simulink model "PEMFuelCellSystem_GasMixture_cEGR_RouteA_v2_v01"  (R2025b)
settings: Solver=VariableStepAuto  StartTime=0.0  StopTime=2500  RelTol=1e-3  AbsTol=1e-3
model workspace: external: MATLAB File E:\agentwork_pemfc_cEGR_0519\04_Simulink物理网络模型\01_模型\RouteA_GasMixture_Derived\PEMFuelCellSystemWithACustomLibraryParameters.m (data not in the file)
undefined symbols (not defined in the file): anode_tube_D, cathode_tube_D, cegr_valve_max_area, cegr_valve_open_min_area, comp_rpm_TLU, coolant_num_layers, coolant_num_passes, coolant_tube_D, coolant_w_channels, env_p, env_T, env_yH20, env_yO2, radiator_air_area_fins, radiator_air_area_primary, radiator_eta_fin, radiator_N_tubes, radiator_rho, radiator_t_wall, radiator_tube_H, radiator_W, routeA_air_pid_Ki, routeA_air_pid_Kp, routeA_anode_source_conditioner_nominal_flow_kg_s, routeA_cathode_source_conditioner_nominal_flow_kg_s, routeA_egr_control_Ki_area, routeA_egr_control_Kp_area, routeA_egr_target_input_mode_id, routeA_egr_valve_actuator_tau, routeA_egr_valve_area_direct, routeA_target_egr_ratio_comp_in, routeA_voltage_current_max_A, routeA_voltage_current_min_A, routeA_voltage_pi_Ki, routeA_voltage_pi_Kp, stack_area, stack_iL, stack_mea_rho, stack_num_cells, stack_num_channels, stack_t_gdl, stack_t_membrane, stack_w_channels, tank_p, tank_T, tank_yH2
libraries: FuelCell_lib x67, fl_lib x67, nesl_utility x56, slpidlib x5
(part 6 of 6)

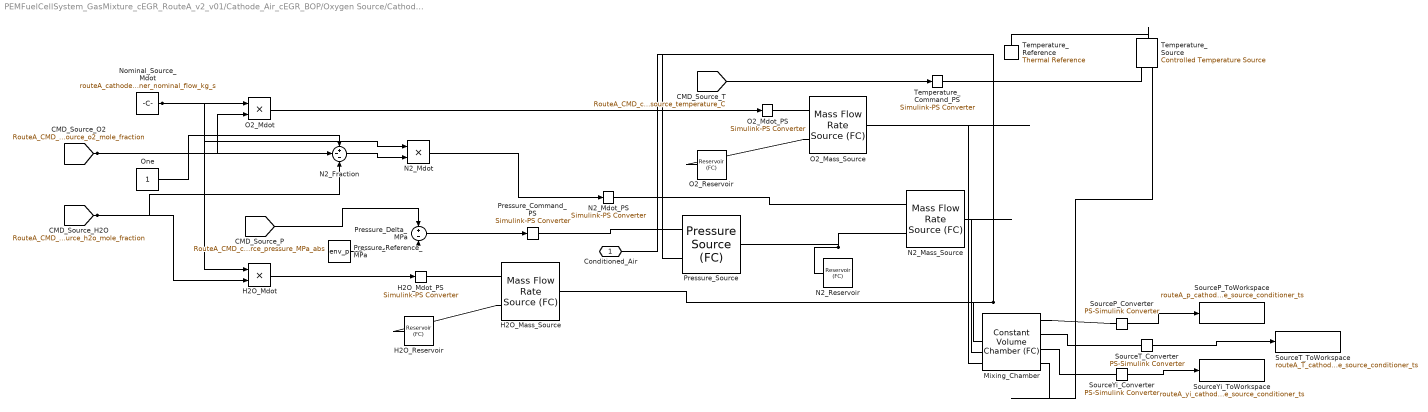
== system PEMFuelCellSystem_GasMixture_cEGR_RouteA_v2_v01/Cathode_Air_cEGR_BOP/Oxygen Source/Cathode_Source_Conditioner ==
  H2O_Mass_Source : FuelCell_lib/sources/Mass Flow Rate Source (FC)  source_type=foundation.enum.constant_controlled.controlled  flow_rate=0 kg/s  power_spec=foundation.enum.power_spec.none  area_A=0.01 m^2  area_B=0.01 m^2  mdot_A_specify=off  mdot_A_priority=None  mdot_A=0.1 kg/s  mdot_A_nominal_specify=off  mdot_A_nominal_value=1  mdot_A_nominal_unit=kg/s  mdot_B_specify=off  mdot_B_priority=None  mdot_B=0.1 kg/s  mdot_B_nominal_specify=off  mdot_B_nominal_value=1  mdot_B_nominal_unit=kg/s  phi_A_specify=off  phi_A_priority=None  phi_A=0 J/s  phi_A_nominal_specify=off  phi_A_nominal_value=1  phi_A_nominal_unit=J/s  phi_B_specify=off  phi_B_priority=None  phi_B=0 J/s  phi_B_nominal_specify=off  phi_B_nominal_value=1  phi_B_nominal_unit=J/s  mdot_A_i_specify=off  mdot_A_i_priority=None  mdot_A_i=[0; 0; 0; 0] kg/s  mdot_A_i_nominal_specify=off  mdot_A_i_nominal_value=1  mdot_A_i_nominal_unit=kg/s  mdot_B_i_specify=off  mdot_B_i_priority=None  mdot_B_i=[0; 0; 0; 0] kg/s  mdot_B_i_nominal_specify=off  mdot_B_i_nominal_value=1  mdot_B_i_nominal_unit=kg/s
      settings: InternalSimscapePortConfiguration="{\"Bottom\":[],\"Left\":[{\"id\":\"M\",\"label\":\"M\",\"type\":\"input\"},{\"id\":\"A\",\"label\":\"A\",\"type\":\"FuelCell.FuelCell\"}],\"Right\":[{\"id\":\"B\",\"label\":\"B\",\"type\":\"FuelCell.FuelCell\"}],\"Top\":[]}"
  H2O_Mdot : Product
  H2O_Mdot_PS : nesl_utility/Simulink-PS Converter  PhysicalDomain=network_engine_domain  SubClassName=ps_input  LeftPortType=input  RightPortType=output  PseudoPeriodic=off  Frequencies=[]  NoiseDistribution=none  NoiseParameters=[]  Unit=kg/s  AffineConversion=off  FilteringAndDerivatives=provide  SimscapeFilterOrder=1  InputFilterTimeConstant=0.001  UdotUserProvided=0
  H2O_Reservoir : FuelCell_lib/elements/Reservoir (FC)  constCond=true  p0=env_p * 1e6 Pa  T0=env_T + 273.15 K  comp=FuelCell.enum.Composition.Mole  y0=[0; 0; 0; 1]  x0=[0; 0; 0; 1]  area=0.01 m^2
      settings: InternalSimscapePortConfiguration="{\"Bottom\":[],\"Left\":[],\"Right\":[],\"Top\":[{\"id\":\"A\",\"label\":\"A\",\"type\":\"FuelCell.FuelCell\"}]}"
  Mixing_Chamber : FuelCell_lib/elements/Constant Volume Chamber (FC)  V0=routeA_cathode_source_conditioner_volume_L l  num_ports=foundation.enum.num_ports.three  area_A=0.01 m^2  area_B=0.01 m^2  area_C=0.01 m^2  area_D=0.01 m^2  cond_spec=FuelCell.enum.ChamberCondSpec.Enabled  tau_c=1 s  is_cond=[0; 0; 0; 1]  out_comp=FuelCell.enum.Composition.Mole  p0=env_p MPa  T0=env_T degC  comp=FuelCell.enum.Composition.Mole  y0=[1-env_yO2-env_yH20; env_yO2; 0; env_yH20]  x0=[1; 0; 0; 0]
      settings: InternalSimscapePortConfiguration="{\"Bottom\":[{\"id\":\"H\",\"label\":\"H\",\"type\":\"foundation.thermal.thermal\"}],\"Left\":[{\"id\":\"MIn\",\"label\":\"MIn\",\"type\":\"input\"},{\"id\":\"TIn\",\"label\":\"TIn\",\"type\":\"input\"}],\"Right\":[{\"id\":\"pC\",\"label\":\"p\",\"type\":\"output\"},{\"id\":\"TC\",\"label\":\"T\",\"type\":\"output\"},{\"id\":\"yC_i\",\"label\":\"y_i\",\"type\":\"output\"}],\"Top\":[{\"id\":\"A\",\"label\":\"A\",\"type\":\"FuelCell.FuelCell\"},{\"id\":\"B\",\"label\":\"B\",\"type\":\"FuelCell.FuelCell\"},{\"id\":\"C\",\"label\":\"C\",\"type\":\"FuelCell.FuelCell\"}]}"
  N2_Fraction : Sum  Inputs=+--
  N2_Mass_Source : FuelCell_lib/sources/Mass Flow Rate Source (FC)  source_type=foundation.enum.constant_controlled.controlled  flow_rate=0 kg/s  power_spec=foundation.enum.power_spec.none  area_A=0.01 m^2  area_B=0.01 m^2  mdot_A_specify=off  mdot_A_priority=None  mdot_A=0.1 kg/s  mdot_A_nominal_specify=off  mdot_A_nominal_value=1  mdot_A_nominal_unit=kg/s  mdot_B_specify=off  mdot_B_priority=None  mdot_B=0.1 kg/s  mdot_B_nominal_specify=off  mdot_B_nominal_value=1  mdot_B_nominal_unit=kg/s  phi_A_specify=off  phi_A_priority=None  phi_A=0 J/s  phi_A_nominal_specify=off  phi_A_nominal_value=1  phi_A_nominal_unit=J/s  phi_B_specify=off  phi_B_priority=None  phi_B=0 J/s  phi_B_nominal_specify=off  phi_B_nominal_value=1  phi_B_nominal_unit=J/s  mdot_A_i_specify=off  mdot_A_i_priority=None  mdot_A_i=[0; 0; 0; 0] kg/s  mdot_A_i_nominal_specify=off  mdot_A_i_nominal_value=1  mdot_A_i_nominal_unit=kg/s  mdot_B_i_specify=off  mdot_B_i_priority=None  mdot_B_i=[0; 0; 0; 0] kg/s  mdot_B_i_nominal_specify=off  mdot_B_i_nominal_value=1  mdot_B_i_nominal_unit=kg/s
      settings: InternalSimscapePortConfiguration="{\"Bottom\":[],\"Left\":[{\"id\":\"M\",\"label\":\"M\",\"type\":\"input\"},{\"id\":\"A\",\"label\":\"A\",\"type\":\"FuelCell.FuelCell\"}],\"Right\":[{\"id\":\"B\",\"label\":\"B\",\"type\":\"FuelCell.FuelCell\"}],\"Top\":[]}"
  N2_Mdot : Product
  N2_Mdot_PS : nesl_utility/Simulink-PS Converter  PhysicalDomain=network_engine_domain  SubClassName=ps_input  LeftPortType=input  RightPortType=output  PseudoPeriodic=off  Frequencies=[]  NoiseDistribution=none  NoiseParameters=[]  Unit=kg/s  AffineConversion=off  FilteringAndDerivatives=provide  SimscapeFilterOrder=1  InputFilterTimeConstant=0.001  UdotUserProvided=0
  N2_Reservoir : FuelCell_lib/elements/Reservoir (FC)  constCond=true  p0=env_p * 1e6 Pa  T0=env_T + 273.15 K  comp=FuelCell.enum.Composition.Mole  y0=[1; 0; 0; 0]  x0=[1; 0; 0; 0]  area=0.01 m^2
      settings: InternalSimscapePortConfiguration="{\"Bottom\":[],\"Left\":[],\"Right\":[],\"Top\":[{\"id\":\"A\",\"label\":\"A\",\"type\":\"FuelCell.FuelCell\"}]}"
  Nominal_Source_Mdot : Constant  Value=routeA_cathode_source_conditioner_nominal_flow_kg_s
  O2_Mass_Source : FuelCell_lib/sources/Mass Flow Rate Source (FC)  source_type=foundation.enum.constant_controlled.controlled  flow_rate=0 kg/s  power_spec=foundation.enum.power_spec.none  area_A=0.01 m^2  area_B=0.01 m^2  mdot_A_specify=off  mdot_A_priority=None  mdot_A=0.1 kg/s  mdot_A_nominal_specify=off  mdot_A_nominal_value=1  mdot_A_nominal_unit=kg/s  mdot_B_specify=off  mdot_B_priority=None  mdot_B=0.1 kg/s  mdot_B_nominal_specify=off  mdot_B_nominal_value=1  mdot_B_nominal_unit=kg/s  phi_A_specify=off  phi_A_priority=None  phi_A=0 J/s  phi_A_nominal_specify=off  phi_A_nominal_value=1  phi_A_nominal_unit=J/s  phi_B_specify=off  phi_B_priority=None  phi_B=0 J/s  phi_B_nominal_specify=off  phi_B_nominal_value=1  phi_B_nominal_unit=J/s  mdot_A_i_specify=off  mdot_A_i_priority=None  mdot_A_i=[0; 0; 0; 0] kg/s  mdot_A_i_nominal_specify=off  mdot_A_i_nominal_value=1  mdot_A_i_nominal_unit=kg/s  mdot_B_i_specify=off  mdot_B_i_priority=None  mdot_B_i=[0; 0; 0; 0] kg/s  mdot_B_i_nominal_specify=off  mdot_B_i_nominal_value=1  mdot_B_i_nominal_unit=kg/s
      settings: InternalSimscapePortConfiguration="{\"Bottom\":[],\"Left\":[{\"id\":\"M\",\"label\":\"M\",\"type\":\"input\"},{\"id\":\"A\",\"label\":\"A\",\"type\":\"FuelCell.FuelCell\"}],\"Right\":[{\"id\":\"B\",\"label\":\"B\",\"type\":\"FuelCell.FuelCell\"}],\"Top\":[]}"
  O2_Mdot : Product
  O2_Mdot_PS : nesl_utility/Simulink-PS Converter  PhysicalDomain=network_engine_domain  SubClassName=ps_input  LeftPortType=input  RightPortType=output  PseudoPeriodic=off  Frequencies=[]  NoiseDistribution=none  NoiseParameters=[]  Unit=kg/s  AffineConversion=off  FilteringAndDerivatives=provide  SimscapeFilterOrder=1  InputFilterTimeConstant=0.001  UdotUserProvided=0
  O2_Reservoir : FuelCell_lib/elements/Reservoir (FC)  constCond=true  p0=env_p * 1e6 Pa  T0=env_T + 273.15 K  comp=FuelCell.enum.Composition.Mole  y0=[0; 1; 0; 0]  x0=[0; 1; 0; 0]  area=0.01 m^2
      settings: InternalSimscapePortConfiguration="{\"Bottom\":[],\"Left\":[],\"Right\":[],\"Top\":[{\"id\":\"A\",\"label\":\"A\",\"type\":\"FuelCell.FuelCell\"}]}"
  One : Constant
  Pressure_Command_PS : nesl_utility/Simulink-PS Converter  PhysicalDomain=network_engine_domain  SubClassName=ps_input  LeftPortType=input  RightPortType=output  PseudoPeriodic=off  Frequencies=[]  NoiseDistribution=none  NoiseParameters=[]  Unit=MPa  AffineConversion=off  FilteringAndDerivatives=filter  SimscapeFilterOrder=1  InputFilterTimeConstant=0.001  UdotUserProvided=0
  Pressure_Delta_MPa : Sum  Inputs=+-
  Pressure_Reference_MPa : Constant  Value=env_p
  Pressure_Source : FuelCell_lib/sources/Pressure Source (FC)  source_type=foundation.enum.constant_controlled.controlled  pressure_differential=0 Pa  power_spec=foundation.enum.power_spec.none  area_A=0.01 m^2  area_B=0.01 m^2  mdot_A_specify=off  mdot_A_priority=None  mdot_A=0.1 kg/s  mdot_A_nominal_specify=off  mdot_A_nominal_value=1  mdot_A_nominal_unit=kg/s  mdot_B_specify=off  mdot_B_priority=None  mdot_B=0.1 kg/s  mdot_B_nominal_specify=off  mdot_B_nominal_value=1  mdot_B_nominal_unit=kg/s  phi_A_specify=off  phi_A_priority=None  phi_A=0 J/s  phi_A_nominal_specify=off  phi_A_nominal_value=1  phi_A_nominal_unit=J/s  phi_B_specify=off  phi_B_priority=None  phi_B=0 J/s  phi_B_nominal_specify=off  phi_B_nominal_value=1  phi_B_nominal_unit=J/s  mdot_A_i_specify=off  mdot_A_i_priority=None  mdot_A_i=[0; 0; 0; 0] kg/s  mdot_A_i_nominal_specify=off  mdot_A_i_nominal_value=1  mdot_A_i_nominal_unit=kg/s  mdot_B_i_specify=off  mdot_B_i_priority=None  mdot_B_i=[0; 0; 0; 0] kg/s  mdot_B_i_nominal_specify=off  mdot_B_i_nominal_value=1  mdot_B_i_nominal_unit=kg/s
      settings: InternalSimscapePortConfiguration="{\"Bottom\":[],\"Left\":[{\"id\":\"p\",\"label\":\"P\",\"type\":\"input\"},{\"id\":\"A\",\"label\":\"A\",\"type\":\"FuelCell.FuelCell\"}],\"Right\":[{\"id\":\"B\",\"label\":\"B\",\"type\":\"FuelCell.FuelCell\"}],\"Top\":[]}"
  SourceP_Converter : nesl_utility/PS-Simulink Converter  PhysicalDomain=network_engine_domain  SubClassName=ps_output  LeftPortType=input  RightPortType=output  PseudoPeriodic=off  Frequencies=[]  VectorFormat=inherit  Unit=inherit  AffineConversion=off
  SourceP_ToWorkspace : ToWorkspace  VariableName=routeA_p_cathode_source_conditioner_ts  SaveFormat=Timeseries  SampleTime=-1
  SourceT_Converter : nesl_utility/PS-Simulink Converter  PhysicalDomain=network_engine_domain  SubClassName=ps_output  LeftPortType=input  RightPortType=output  PseudoPeriodic=off  Frequencies=[]  VectorFormat=inherit  Unit=inherit  AffineConversion=off
  SourceT_ToWorkspace : ToWorkspace  VariableName=routeA_T_cathode_source_conditioner_ts  SaveFormat=Timeseries  SampleTime=-1
  SourceYi_Converter : nesl_utility/PS-Simulink Converter  PhysicalDomain=network_engine_domain  SubClassName=ps_output  LeftPortType=input  RightPortType=output  PseudoPeriodic=off  Frequencies=[]  VectorFormat=inherit  Unit=inherit  AffineConversion=off
  SourceYi_ToWorkspace : ToWorkspace  VariableName=routeA_yi_cathode_source_conditioner_ts  SaveFormat=Timeseries  SampleTime=-1
  Temperature_Command_PS : nesl_utility/Simulink-PS Converter  PhysicalDomain=network_engine_domain  SubClassName=ps_input  LeftPortType=input  RightPortType=output  PseudoPeriodic=off  Frequencies=[]  NoiseDistribution=none  NoiseParameters=[]  Unit=degC  AffineConversion=off  FilteringAndDerivatives=filter  SimscapeFilterOrder=1  InputFilterTimeConstant=0.001  UdotUserProvided=0
  Temperature_Reference : fl_lib/Thermal/Thermal Elements/Thermal Reference
  Temperature_Source : fl_lib/Thermal/Thermal Sources/Controlled Temperature Source
  Conditioned_Air : PMIOPort  Side=Right
  wires:
  SourceYi_Converter/1 -> SourceYi_ToWorkspace/1
  SourceT_Converter/1 -> SourceT_ToWorkspace/1
  Pressure_Delta_MPa/1 -> Pressure_Command_PS/1
  Pressure_Reference_MPa/1 -> Pressure_Delta_MPa/2
  [RouteA_CMD_cathode_source_pressure_MPa_abs] -> Pressure_Delta_MPa/1
  [RouteA_CMD_cathode_source_temperature_C] -> Temperature_Command_PS/1
  One/1 -> N2_Fraction/1
  [RouteA_CMD_cathode_source_o2_mole_fraction] -> O2_Mdot/2, N2_Fraction/2
  [RouteA_CMD_cathode_source_h2o_mole_fraction] -> N2_Fraction/3, H2O_Mdot/2
  Nominal_Source_Mdot/1 -> O2_Mdot/1, N2_Mdot/1, H2O_Mdot/1
  N2_Fraction/1 -> N2_Mdot/2
  N2_Mdot/1 -> N2_Mdot_PS/1
  O2_Mdot/1 -> O2_Mdot_PS/1
  H2O_Mdot/1 -> H2O_Mdot_PS/1
  SourceP_Converter/1 -> SourceP_ToWorkspace/1
  connections:
  Mixing_Chamber/RConn3 -- SourceYi_Converter/LConn1
  Mixing_Chamber/RConn2 -- SourceT_Converter/LConn1
  Pressure_Command_PS/RConn1 -- Pressure_Source/LConn1
  Mixing_Chamber/LConn3 -- H2O_Mass_Source/RConn1 -- Pressure_Source/LConn2 -- Conditioned_Air/RConn1
  Temperature_Command_PS/RConn1 -- Temperature_Source/RConn1
  Temperature_Source/RConn2 -- Mixing_Chamber/RConn4
  Temperature_Source/LConn1 -- Temperature_Reference/LConn1
  N2_Mdot_PS/RConn1 -- N2_Mass_Source/LConn1
  O2_Mdot_PS/RConn1 -- O2_Mass_Source/LConn1
  H2O_Mdot_PS/RConn1 -- H2O_Mass_Source/LConn1
  N2_Reservoir/LConn1 -- Pressure_Source/RConn1 -- N2_Mass_Source/LConn2
  O2_Reservoir/LConn1 -- O2_Mass_Source/LConn2
  H2O_Reservoir/LConn1 -- H2O_Mass_Source/LConn2
  N2_Mass_Source/RConn1 -- Mixing_Chamber/LConn4
  O2_Mass_Source/RConn1 -- Mixing_Chamber/LConn5
  Mixing_Chamber/RConn1 -- SourceP_Converter/LConn1

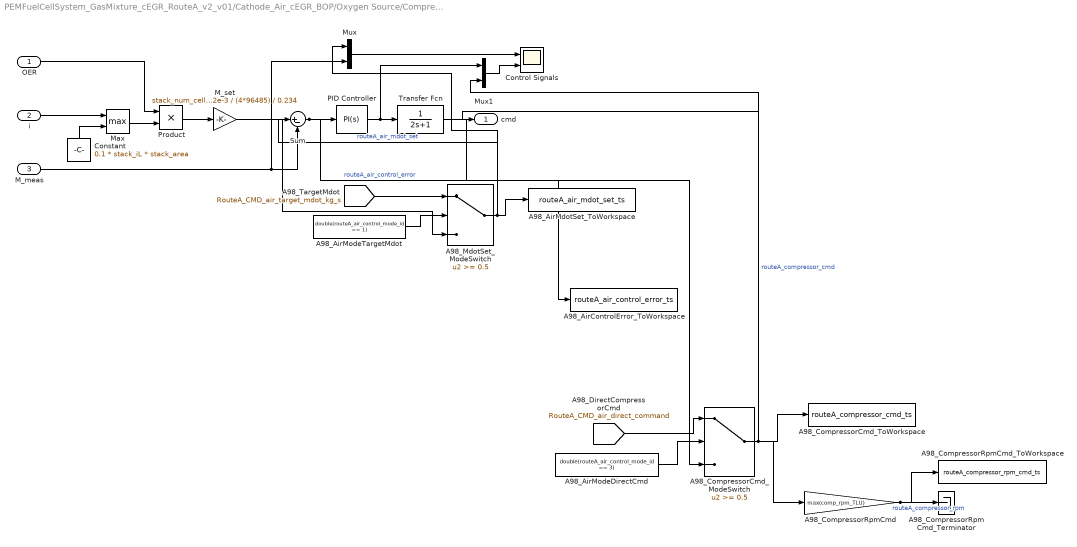
== system PEMFuelCellSystem_GasMixture_cEGR_RouteA_v2_v01/Cathode_Air_cEGR_BOP/Oxygen Source/Compressor Control ==
  OER : Inport
  i : Inport  Port=2
  M_meas : Inport  Port=3
  A98_AirControlError_ToWorkspace : ToWorkspace  VariableName=routeA_air_control_error_ts  SaveFormat=Timeseries  SampleTime=-1
  A98_AirMdotSet_ToWorkspace : ToWorkspace  VariableName=routeA_air_mdot_set_ts  SaveFormat=Timeseries  SampleTime=-1
  A98_AirModeDirectCmd : Constant  Value=double(routeA_air_control_mode_id == 3)
  A98_AirModeTargetMdot : Constant  Value=double(routeA_air_control_mode_id == 1)
  A98_CompressorCmd_ModeSwitch : Switch  Threshold=0.5  SaturateOnIntegerOverflow=off  InputSameDT=off
  A98_CompressorCmd_ToWorkspace : ToWorkspace  VariableName=routeA_compressor_cmd_ts  SaveFormat=Timeseries  SampleTime=-1
  A98_CompressorRpmCmd : Gain  Gain=max(comp_rpm_TLU)
  A98_CompressorRpmCmd_Terminator : Terminator
  A98_CompressorRpmCmd_ToWorkspace : ToWorkspace  VariableName=routeA_compressor_rpm_cmd_ts  SaveFormat=Timeseries  SampleTime=-1
  A98_MdotSet_ModeSwitch : Switch  Threshold=0.5  SaturateOnIntegerOverflow=off  InputSameDT=off
  Constant : Constant  Value=0.1 * stack_iL * stack_area
  Control Signals : Scope  NumInputPorts=2
      settings: Title=Mass Flow Rate (kg/s)  ActiveDisplayYMinimum=-0.01736  ActiveDisplayYMaximum=0.15625  DataLoggingVariableName=ScopeData2
  M_set : Gain  Gain=stack_num_cells * 32e-3 / (4*96485) / 0.234
  Max : MinMax  Function=max  Inputs=2  ZeroCross=off
  Mux : Mux  Inputs=2
  Mux1 : Mux  Inputs=2
  PID Controller : slpidlib/PID Controller  Controller=PI  Form=Ideal  TimeDomain=Continuous-time  UseExternalTs=off  SampleTime=-1  IntegratorMethod=Forward Euler  FilterMethod=Forward Euler  ControllerParametersSource=internal  P=routeA_air_pid_Kp  I=routeA_air_pid_Ki  UseKiTs=off  D=0  UseExternalDerivativeSource=off  N=100  UseFilter=on  TunerSelectOption=Transfer Function Based (PID Tuner App)  InitialConditionSource=internal  InitialConditionForIntegrator=0  InitialConditionForFilter=0  DifferentiatorICPrevScaledInput=0  ExternalReset=none  TrackingMode=off  Kt=1  LimitOutput=on  SatLimitsSource=internal  UpperSaturationLimit=1  LowerSaturationLimit=0  LinearizeAsGain=on  AntiWindupMode=back-calculation  Kb=1  LimitIntegrator=off  UpperIntegratorSaturationLimit=inf  LowerIntegratorSaturationLimit=-inf  POutMin=[]  POutMax=[]  IOutMin=[]  IOutMax=[]  DOutMin=[]  DOutMax=[]  NOutMin=[]  NOutMax=[]  SumOutMin=[]  SumOutMax=[]  SaturationOutMin=[]  SaturationOutMax=[]  PParamMin=[]  PParamMax=[]  IParamMin=[]  IParamMax=[]  DParamMin=[]  DParamMax=[]  NParamMin=[]  NParamMax=[]  KbParamMin=[]  KbParamMax=[]  KtParamMin=[]  KtParamMax=[]  KbOutMin=[]  KbOutMax=[]  KtOutMin=[]  KtOutMax=[]  IntegratorOutMin=[]  IntegratorOutMax=[]  FilterOutMin=[]  FilterOutMax=[]  SumI1OutMin=[]  SumI1OutMax=[]  SumI2OutMin=[]  SumI2OutMax=[]  SumI3OutMin=[]  SumI3OutMax=[]  SumI4OutMin=[]  SumI4OutMax=[]  SumDOutMin=[]  SumDOutMax=[]  DifferentiatorOutMin=[]  DifferentiatorOutMax=[]  FilterDiffOutCoefMin=[]  FilterDiffOutCoefMax=[]  ReciprocalOutMin=[]  ReciprocalOutMax=[]  SumDenOutMin=[]  SumDenOutMax=[]  SumNumOutMin=[]  SumNumOutMax=[]  DivideOutMin=[]  DivideOutMax=[]  UdiffTsProdOutMin=[]  UdiffTsProdOutMax=[]  NTsProdOutMin=[]  NTsProdOutMax=[]  UintegralTsProdOutMin=[]  UintegralTsProdOutMax=[]  UngainTsProdOutMin=[]  UngainTsProdOutMax=[]  ClampingZeroOutDataTypeStr=Inherit: Inherit via back propagation  ClampingZeroOutMin=[]  ClampingZeroOutMax=[]  FilterDenConstantOutDataTypeStr=Inherit: Inherit via back propagation  FilterDenConstantOutMin=[]  FilterDenConstantOutMax=[]  PCopyOutDataTypeStr=Inherit: Inherit via back propagation  PCopyOutMin=[]  PCopyOutMax=[]  NCopyOutDataTypeStr=Inherit: Inherit via back propagation  NCopyOutMin=[]  NCopyOutMax=[]  IntegratorContinuousStateAttributes=''  IntegratorStateMustResolveToSignalObject=off  IntegratorRTWStateStorageClass=Auto  FilterContinuousStateAttributes=''  FilterStateMustResolveToSignalObject=off  FilterRTWStateStorageClass=Auto  ParallelPVariant=Passthrough  IdealPVariant=InternalParameters  IVariant=InternalParameters  DVariant=Disabled  IntegratorVariant=Continuous  SatVariant=Enabled  AWVariant=BackCalculation  PCopyVariant=Disabled  TRVariant=Disabled  FdbkBlocksVariant=Forward  IdealPFdbkVariant=Disabled  SatFdbkVariant=Disabled  DerivativeFilterVariant=Disabled  NVariant=Disabled  NCopyVariant=Disabled_SignalSpec  FilterICVariant=Disabled  IntegratorICVariant=InternalICs  ExternalResetVariant=Disabled  TRSumVariant=Passthrough  SumFdbkVariant=Disabled  SumVariant=Sum_PI  TsampFilterVariant=InternalTs  TsampNgainVariant=Passthrough  TsampIntegralVariant=Disabled_SignalSpec  ExternalSaturationOutDataTypeStr=Inherit: Same as second input  DerivativeSourceVariant=Disabled  PreIntVariant=InternalPreInt
  Product : Product
  Sum : Sum  Inputs=|+-
  Transfer Fcn : TransferFcn  Denominator=[2 1]
  cmd : Outport
  wires:
  OER/1 -> Product/1
  Constant/1 -> Max/2
  i/1 -> Max/1
  Max/1 -> Product/2
  PID Controller/1 -> Mux1/1, Transfer Fcn/1
  Sum/1 -> PID Controller/1, A98_AirControlError_ToWorkspace/1  "routeA_air_control_error"
  Product/1 -> M_set/1
  M_meas/1 -> Mux/2, Sum/2
  Mux/1 -> Control Signals/1
  Mux1/1 -> Control Signals/2
  A98_AirModeTargetMdot/1 -> A98_MdotSet_ModeSwitch/2
  M_set/1 -> A98_MdotSet_ModeSwitch/3
  A98_MdotSet_ModeSwitch/1 -> Sum/1, Mux/1, A98_AirMdotSet_ToWorkspace/1  "routeA_air_mdot_set"
  A98_AirModeDirectCmd/1 -> A98_CompressorCmd_ModeSwitch/2
  Transfer Fcn/1 -> A98_CompressorCmd_ModeSwitch/3
  A98_CompressorCmd_ModeSwitch/1 -> cmd/1, Mux1/2, A98_CompressorRpmCmd/1, A98_CompressorCmd_ToWorkspace/1  "routeA_compressor_cmd"
  A98_CompressorRpmCmd/1 -> A98_CompressorRpmCmd_Terminator/1, A98_CompressorRpmCmd_ToWorkspace/1  "routeA_compressor_rpm"
  [RouteA_CMD_air_target_mdot_kg_s] -> A98_MdotSet_ModeSwitch/1
  [RouteA_CMD_air_direct_command] -> A98_CompressorCmd_ModeSwitch/1

== system PEMFuelCellSystem_GasMixture_cEGR_RouteA_v2_v01/Cathode_Air_cEGR_BOP/Oxygen Source/Compressor Map ==
  1 / 101325 : fl_lib/Physical Signals/Functions/PS Gain  gain=1 / 101325 1/Pa
  1 / 288.15 : fl_lib/Physical Signals/Functions/PS Gain  gain=1 / 288.15 1/K
  Absolute Reference (FC) : FuelCell_lib/elements/Absolute Reference (FC)
      settings: InternalSimscapePortConfiguration="{\"Bottom\":[],\"Left\":[{\"id\":\"A\",\"label\":\"\",\"type\":\"FuelCell.FuelCell\"}],\"Right\":[],\"Top\":[]}"
  Absolute Reference (FC)1 : FuelCell_lib/elements/Absolute Reference (FC)
      settings: InternalSimscapePortConfiguration="{\"Bottom\":[],\"Left\":[{\"id\":\"A\",\"label\":\"\",\"type\":\"FuelCell.FuelCell\"}],\"Right\":[],\"Top\":[]}"
  Corrected Flow Table : fl_lib/Physical Signals/Lookup Tables/PS Lookup Table (2D)  x1=comp_p_ratio_TLU Pa/Pa  x2=comp_rpm_TLU rpm  f=comp_mdot_corr_TLU kg/s  interp_method=simscape.enum.interpolation.linear  extrap_method=simscape.enum.extrapolation.nearest
  PS Divide : fl_lib/Physical Signals/Functions/PS Divide
  PS Divide1 : fl_lib/Physical Signals/Functions/PS Divide
  PS Product : fl_lib/Physical Signals/Functions/PS Product
  Pressure and Temperature Sensor (FC) : FuelCell_lib/sensors/Pressure and Temperature Sensor (FC)
      settings: InternalSimscapePortConfiguration="{\"Bottom\":[],\"Left\":[{\"id\":\"A\",\"label\":\"A\",\"type\":\"FuelCell.FuelCell\"}],\"Right\":[{\"id\":\"P\",\"label\":\"P\",\"type\":\"output\"},{\"id\":\"T\",\"label\":\"T\",\"type\":\"output\"},{\"id\":\"B\",\"label\":\"B\",\"type\":\"FuelCell.FuelCell\"}],\"Top\":[]}"
  Pressure and Temperature Sensor (FC)1 : FuelCell_lib/sensors/Pressure and Temperature Sensor (FC)
      settings: InternalSimscapePortConfiguration="{\"Bottom\":[],\"Left\":[{\"id\":\"A\",\"label\":\"A\",\"type\":\"FuelCell.FuelCell\"}],\"Right\":[{\"id\":\"P\",\"label\":\"P\",\"type\":\"output\"},{\"id\":\"T\",\"label\":\"T\",\"type\":\"output\"},{\"id\":\"B\",\"label\":\"B\",\"type\":\"FuelCell.FuelCell\"}],\"Top\":[]}"
  TDenGuardBias : fl_lib/Physical Signals/Functions/PS Bias  bias=cegr_comp_map_t_denom_epsilon
      settings: InternalSimscapePortConfiguration="{\"Bottom\":[],\"Left\":[{\"id\":\"I\",\"label\":\"\",\"type\":\"input\"}],\"Right\":[{\"id\":\"O\",\"label\":\"\",\"type\":\"output\"}],\"Top\":[]}"
  sqrt : fl_lib/Physical Signals/Functions/PS Math Function  fcn_choice=foundation.enum.math_function.sqrt  v=1
  mdot : PMIOPort  Side=Left
  in : PMIOPort  Port=2  Side=Right
  rpm : PMIOPort  Port=3  Side=Right
  out : PMIOPort  Port=4  Side=Right
  connections:
  1 / 101325/LConn1 -- Pressure and Temperature Sensor (FC)/RConn1 -- PS Divide/LConn2
  rpm/RConn1 -- Corrected Flow Table/LConn2
  PS Divide/RConn1 -- Corrected Flow Table/LConn1
  1 / 288.15/LConn1 -- Pressure and Temperature Sensor (FC)/RConn2
  PS Product/LConn1 -- 1 / 101325/RConn1
  PS Product/LConn2 -- Corrected Flow Table/RConn1
  PS Divide1/LConn1 -- PS Product/RConn1
  1 / 288.15/RConn1 -- sqrt/LConn1
  mdot/RConn1 -- PS Divide1/RConn1
  Pressure and Temperature Sensor (FC)1/RConn1 -- PS Divide/LConn1
  Absolute Reference (FC)/LConn1 -- Pressure and Temperature Sensor (FC)/RConn3
  Pressure and Temperature Sensor (FC)/LConn1 -- in/RConn1
  Absolute Reference (FC)1/LConn1 -- Pressure and Temperature Sensor (FC)1/RConn3
  Pressure and Temperature Sensor (FC)1/LConn1 -- out/RConn1
  sqrt/RConn1 -- TDenGuardBias/LConn1
  TDenGuardBias/RConn1 -- PS Divide1/LConn2

== system PEMFuelCellSystem_GasMixture_cEGR_RouteA_v2_v01/Cathode_Exhaust_Backpressure_Water/Cathode Exhaust/Pressure Relief Valve ==
  Absolute Reference (FC) : FuelCell_lib/elements/Absolute Reference (FC)
      settings: InternalSimscapePortConfiguration="{\"Bottom\":[],\"Left\":[{\"id\":\"A\",\"label\":\"\",\"type\":\"FuelCell.FuelCell\"}],\"Right\":[],\"Top\":[]}"
  PS Add : fl_lib/Physical Signals/Functions/PS Add
  PS Constant : fl_lib/Physical Signals/Sources/PS Constant  constant=r_min^2
  PS Gain : fl_lib/Physical Signals/Functions/PS Gain  gain=(r_max^2 - r_min^2)/p_range 1/MPa
  PS Gain1 : fl_lib/Physical Signals/Functions/PS Gain  gain=pi*D^2/4 m^2
  PS Subtract : fl_lib/Physical Signals/Functions/PS Subtract
  Pressure and Temperature Sensor (FC) : FuelCell_lib/sensors/Pressure and Temperature Sensor (FC)
      settings: InternalSimscapePortConfiguration="{\"Bottom\":[],\"Left\":[{\"id\":\"A\",\"label\":\"A\",\"type\":\"FuelCell.FuelCell\"}],\"Right\":[{\"id\":\"P\",\"label\":\"P\",\"type\":\"output\"},{\"id\":\"T\",\"label\":\"T\",\"type\":\"output\"},{\"id\":\"B\",\"label\":\"B\",\"type\":\"FuelCell.FuelCell\"}],\"Top\":[]}"
  Valve : FuelCell_lib/elements/Local Restriction (FC)  const_area=false  restriction_area=0.001 m^2  min_area=pi*(r_min*D)^2/4 m^2  max_area=pi*(r_max*D)^2/4 m^2  area=pi*D^2/4 m^2  Cd=0.64  B_lam=0.999
      settings: InternalSimscapePortConfiguration="{\"Bottom\":[],\"Left\":[{\"id\":\"AR\",\"label\":\"AR\",\"type\":\"input\"},{\"id\":\"A\",\"label\":\"A\",\"type\":\"FuelCell.FuelCell\"}],\"Right\":[{\"id\":\"B\",\"label\":\"B\",\"type\":\"FuelCell.FuelCell\"}],\"Top\":[]}"
  A : PMIOPort  Side=Left
  B : PMIOPort  Port=2  Side=Right
  p_set : PMIOPort  Port=3  Side=Left
  connections:
  PS Add/RConn1 -- PS Gain1/LConn1
  PS Gain/LConn1 -- PS Subtract/RConn1
  PS Gain1/RConn1 -- Valve/LConn1
  Valve/RConn1 -- B/RConn1
  A/RConn1 -- Pressure and Temperature Sensor (FC)/LConn1 -- Valve/LConn2
  PS Gain/RConn1 -- PS Add/LConn1
  PS Add/LConn2 -- PS Constant/RConn1
  p_set/RConn1 -- PS Subtract/LConn2
  Pressure and Temperature Sensor (FC)/RConn1 -- PS Subtract/LConn1
  Absolute Reference (FC)/LConn1 -- Pressure and Temperature Sensor (FC)/RConn3

== system PEMFuelCellSystem_GasMixture_cEGR_RouteA_v2_v01/System_Control_Observability/Electrical Load/Inputs ==
  Current Demand : Subsystem  VariantControl=Current
      settings: PortSchema="{\"entries\":[{\"content\":{\"sides\":[{\"content\":{\"connectorIds\":[\"LConn1\"]},\"type\":\"ConnectorPlacement.EquallySpacedRectSide\",\"uuid\":\"316ab41f-9548-4c29-941b-82cd3006a9cc\"},{\"content\":{\"connectorIds\":[],\"side\":\"RIGHT\"},\"type\":\"ConnectorPlacement.EquallySpacedRectSide\",\"uuid\":\"21ddf6a1-5f8a-47a4-ab15-3c27c3a556ce\"},{\"content\":{\"connectorIds\":[\"LConn2\"],\"side\":\"TOP\"},\"type\":\"ConnectorPlacement.EquallySpacedRectSide\",\"uuid\":\"59191a52-f145-4ac2-9cf2-0e0b54b3d2a8\"}]},\"type\":\"ConnectorPlacement.EquallySpacedConnector\",\"uuid\":\"e8f988fd-b412-4b1a-aaea-374cf82170cc\"}],\"packageUris\":[\"http://schema.mathworks.com/mf0/Connector/R2020b\"],\"version\":\"1.0\"}"
      mask Display:
      | plot(0, 0)
      | plot(100, 100)
      | 
      | plot([20 50 50 80], [20 20 80 80])
  Power Demand : Subsystem  VariantControl=Power
      settings: PortSchema="{\"entries\":[{\"content\":{\"sides\":[{\"content\":{\"connectorIds\":[\"LConn1\"]},\"type\":\"ConnectorPlacement.EquallySpacedRectSide\",\"uuid\":\"316ab41f-9548-4c29-941b-82cd3006a9cc\"},{\"content\":{\"connectorIds\":[],\"side\":\"RIGHT\"},\"type\":\"ConnectorPlacement.EquallySpacedRectSide\",\"uuid\":\"21ddf6a1-5f8a-47a4-ab15-3c27c3a556ce\"},{\"content\":{\"connectorIds\":[\"LConn2\"],\"side\":\"TOP\"},\"type\":\"ConnectorPlacement.EquallySpacedRectSide\",\"uuid\":\"59191a52-f145-4ac2-9cf2-0e0b54b3d2a8\"}]},\"type\":\"ConnectorPlacement.EquallySpacedConnector\",\"uuid\":\"e8f988fd-b412-4b1a-aaea-374cf82170cc\"}],\"packageUris\":[\"http://schema.mathworks.com/mf0/Connector/R2020b\"],\"version\":\"1.0\"}"
      mask Display:
      | plot(0, 0)
      | plot(100, 100)
      | 
      | mws = get_param(bdroot, 'ModelWorkspace');
      | x = getVariable(mws, 'drive_cycle_time');
      | y = getVariable(mws, 'drive_cycle_power');
      | 
      | plot(x/max(x)*80 + 10, y/max(y)*60 + 30)
  Voltage Demand : Subsystem  VariantControl=Voltage
  i : PMIOPort  Side=Left
  v : PMIOPort  Port=2  Side=Left

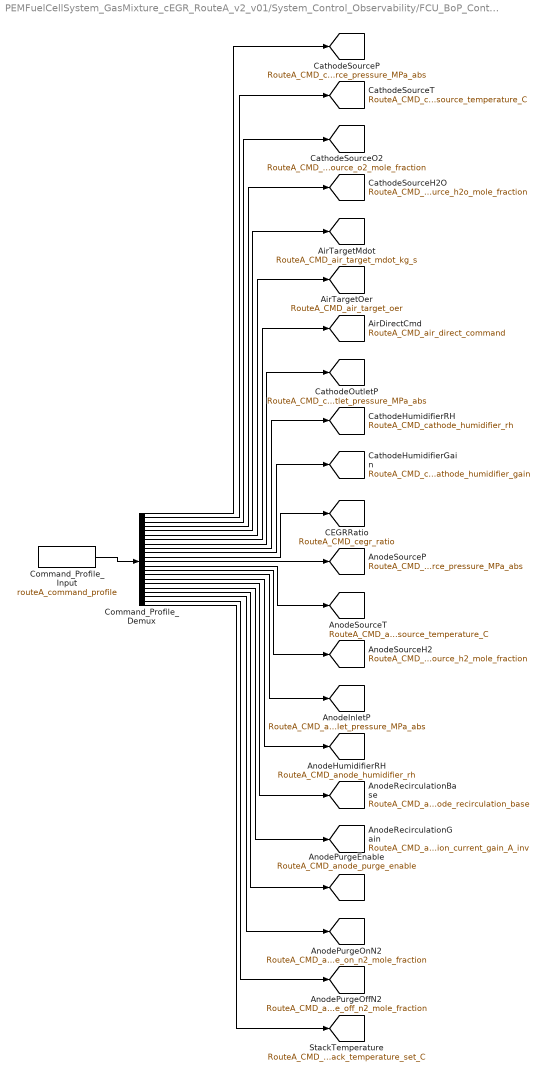
== system PEMFuelCellSystem_GasMixture_cEGR_RouteA_v2_v01/System_Control_Observability/FCU_BoP_Control/RouteA_Command_Profile ==
  Command_Profile_Demux : Demux  Outputs=22
  Command_Profile_Input : FromWorkspace  VariableName=routeA_command_profile  OutputAfterFinalValue=Holding final value
  tag scope: RouteA_CMD_air_direct_command=global, RouteA_CMD_air_target_mdot_kg_s=global, RouteA_CMD_air_target_oer=global, RouteA_CMD_anode_humidifier_rh=global, RouteA_CMD_anode_inlet_pressure_MPa_abs=global, RouteA_CMD_anode_purge_enable=global, RouteA_CMD_anode_purge_off_n2_mole_fraction=global, RouteA_CMD_anode_purge_on_n2_mole_fraction=global, RouteA_CMD_anode_recirculation_base=global, RouteA_CMD_anode_recirculation_current_gain_A_inv=global, RouteA_CMD_anode_source_h2_mole_fraction=global, RouteA_CMD_anode_source_pressure_MPa_abs=global, RouteA_CMD_anode_source_temperature_C=global, RouteA_CMD_cathode_humidifier_gain=global, RouteA_CMD_cathode_humidifier_rh=global, RouteA_CMD_cathode_outlet_pressure_MPa_abs=global, RouteA_CMD_cathode_source_h2o_mole_fraction=global, RouteA_CMD_cathode_source_o2_mole_fraction=global, RouteA_CMD_cathode_source_pressure_MPa_abs=global, RouteA_CMD_cathode_source_temperature_C=global, RouteA_CMD_cegr_ratio=global, RouteA_CMD_stack_temperature_set_C=global
  wires:
  Command_Profile_Demux/22 -> [RouteA_CMD_stack_temperature_set_C]
  Command_Profile_Demux/21 -> [RouteA_CMD_anode_purge_off_n2_mole_fraction]
  Command_Profile_Demux/20 -> [RouteA_CMD_anode_purge_on_n2_mole_fraction]
  Command_Profile_Demux/19 -> [RouteA_CMD_anode_purge_enable]
  Command_Profile_Demux/18 -> [RouteA_CMD_anode_recirculation_current_gain_A_inv]
  Command_Profile_Demux/17 -> [RouteA_CMD_anode_recirculation_base]
  Command_Profile_Demux/16 -> [RouteA_CMD_anode_humidifier_rh]
  Command_Profile_Demux/15 -> [RouteA_CMD_anode_inlet_pressure_MPa_abs]
  Command_Profile_Demux/14 -> [RouteA_CMD_anode_source_h2_mole_fraction]
  Command_Profile_Demux/13 -> [RouteA_CMD_anode_source_temperature_C]
  Command_Profile_Demux/12 -> [RouteA_CMD_anode_source_pressure_MPa_abs]
  Command_Profile_Demux/11 -> [RouteA_CMD_cegr_ratio]
  Command_Profile_Demux/10 -> [RouteA_CMD_cathode_humidifier_gain]
  Command_Profile_Demux/9 -> [RouteA_CMD_cathode_humidifier_rh]
  Command_Profile_Demux/8 -> [RouteA_CMD_cathode_outlet_pressure_MPa_abs]
  Command_Profile_Demux/7 -> [RouteA_CMD_air_direct_command]
  Command_Profile_Demux/6 -> [RouteA_CMD_air_target_oer]
  Command_Profile_Demux/5 -> [RouteA_CMD_air_target_mdot_kg_s]
  Command_Profile_Demux/4 -> [RouteA_CMD_cathode_source_h2o_mole_fraction]
  Command_Profile_Demux/3 -> [RouteA_CMD_cathode_source_o2_mole_fraction]
  Command_Profile_Demux/2 -> [RouteA_CMD_cathode_source_temperature_C]
  Command_Profile_Demux/1 -> [RouteA_CMD_cathode_source_pressure_MPa_abs]
  Command_Profile_Input/1 -> Command_Profile_Demux/1

== system PEMFuelCellSystem_GasMixture_cEGR_RouteA_v2_v01/Thermal_Management_BOP/Cooling System/Coolant Tank ==
  Coolant Volume : fl_lib/Thermal Liquid/Elements/Translational Mechanical Converter (TL)  mech_orientation=foundation.enum.MechOrientationTranslational.Positive  displacement_spec=foundation.enum.DisplacementSpec.Calculate  x0=x_init m  interface_area=A m^2  dead_volume=A * 0.001 m^3  environment_spec=foundation.enum.pressure_spec.atmospheric  environment_pressure=0.101325 MPa  dynamic_compressibility=simscape.enum.onoff.off  p0=env_p MPa  T0=env_T degC  p_nominal=0.101325 MPa  T_nominal=293.15 K
      settings: InternalSimscapePortConfiguration="{\"Bottom\":[],\"Left\":[{\"id\":\"A\",\"label\":\"A\",\"type\":\"foundation.thermal_liquid.thermal_liquid\"},{\"id\":\"C\",\"label\":\"C\",\"type\":\"foundation.mechanical.translational.translational\"},{\"id\":\"H\",\"label\":\"H\",\"type\":\"foundation.thermal.thermal\"}],\"Right\":[{\"id\":\"R\",\"label\":\"R\",\"type\":\"foundation.mechanical.translational.translational\"}],\"Top\":[]}"
  Mechanical Translational Reference : fl_lib/Mechanical/Translational Elements/Mechanical Translational Reference
  Perfect Insulator : fl_lib/Thermal/Thermal Elements/Perfect Insulator  T_specify=off  T_priority=None  T=0 K  T_nominal_specify=off  T_nominal_value=1  T_nominal_unit=K
  Translational Free End : fl_lib/Mechanical/Translational Elements/Translational Free End  v_specify=off  v_priority=None  v=0 m/s  v_nominal_specify=off  v_nominal_value=1  v_nominal_unit=m/s
      settings: InternalSimscapePortConfiguration="{\"Bottom\":[],\"Left\":[{\"id\":\"V\",\"label\":\"\",\"type\":\"foundation.mechanical.translational.translational\"}],\"Right\":[],\"Top\":[]}"
  T : PMIOPort  Side=Right
  connections:
  Coolant Volume/LConn1 -- T/RConn1
  Mechanical Translational Reference/LConn1 -- Coolant Volume/LConn2
  Translational Free End/LConn1 -- Coolant Volume/RConn1
  Perfect Insulator/LConn1 -- Coolant Volume/LConn3

== system PEMFuelCellSystem_GasMixture_cEGR_RouteA_v2_v01/Thermal_Management_BOP/Cooling System/Pump Control ==
  T_set : Inport
  T_meas : Inport  Port=2
  Control Signals : Scope  NumInputPorts=2
      settings: Title=Stack Temperature (degC)  ActiveDisplayYMinimum=12.33618  ActiveDisplayYMaximum=88.97437
  Mux : Mux  Inputs=2
  Mux1 : Mux  Inputs=2
  PID Controller : slpidlib/PID Controller  Controller=PI  Form=Ideal  TimeDomain=Continuous-time  UseExternalTs=off  SampleTime=-1  IntegratorMethod=Forward Euler  FilterMethod=Forward Euler  ControllerParametersSource=internal  P=0.1  I=0.01  UseKiTs=off  D=0  UseExternalDerivativeSource=off  N=100  UseFilter=on  TunerSelectOption=Transfer Function Based (PID Tuner App)  InitialConditionSource=internal  InitialConditionForIntegrator=0  InitialConditionForFilter=0  DifferentiatorICPrevScaledInput=0  ExternalReset=none  TrackingMode=off  Kt=1  LimitOutput=on  SatLimitsSource=internal  UpperSaturationLimit=1  LowerSaturationLimit=0  LinearizeAsGain=on  AntiWindupMode=back-calculation  Kb=0.1  LimitIntegrator=off  UpperIntegratorSaturationLimit=inf  LowerIntegratorSaturationLimit=-inf  POutMin=[]  POutMax=[]  IOutMin=[]  IOutMax=[]  DOutMin=[]  DOutMax=[]  NOutMin=[]  NOutMax=[]  SumOutMin=[]  SumOutMax=[]  SaturationOutMin=[]  SaturationOutMax=[]  PParamMin=[]  PParamMax=[]  IParamMin=[]  IParamMax=[]  DParamMin=[]  DParamMax=[]  NParamMin=[]  NParamMax=[]  KbParamMin=[]  KbParamMax=[]  KtParamMin=[]  KtParamMax=[]  KbOutMin=[]  KbOutMax=[]  KtOutMin=[]  KtOutMax=[]  IntegratorOutMin=[]  IntegratorOutMax=[]  FilterOutMin=[]  FilterOutMax=[]  SumI1OutMin=[]  SumI1OutMax=[]  SumI2OutMin=[]  SumI2OutMax=[]  SumI3OutMin=[]  SumI3OutMax=[]  SumI4OutMin=[]  SumI4OutMax=[]  SumDOutMin=[]  SumDOutMax=[]  DifferentiatorOutMin=[]  DifferentiatorOutMax=[]  FilterDiffOutCoefMin=[]  FilterDiffOutCoefMax=[]  ReciprocalOutMin=[]  ReciprocalOutMax=[]  SumDenOutMin=[]  SumDenOutMax=[]  SumNumOutMin=[]  SumNumOutMax=[]  DivideOutMin=[]  DivideOutMax=[]  UdiffTsProdOutMin=[]  UdiffTsProdOutMax=[]  NTsProdOutMin=[]  NTsProdOutMax=[]  UintegralTsProdOutMin=[]  UintegralTsProdOutMax=[]  UngainTsProdOutMin=[]  UngainTsProdOutMax=[]  ClampingZeroOutDataTypeStr=Inherit: Inherit via back propagation  ClampingZeroOutMin=[]  ClampingZeroOutMax=[]  FilterDenConstantOutDataTypeStr=Inherit: Inherit via back propagation  FilterDenConstantOutMin=[]  FilterDenConstantOutMax=[]  PCopyOutDataTypeStr=Inherit: Inherit via back propagation  PCopyOutMin=[]  PCopyOutMax=[]  NCopyOutDataTypeStr=Inherit: Inherit via back propagation  NCopyOutMin=[]  NCopyOutMax=[]  IntegratorContinuousStateAttributes=''  IntegratorStateMustResolveToSignalObject=off  IntegratorRTWStateStorageClass=Auto  FilterContinuousStateAttributes=''  FilterStateMustResolveToSignalObject=off  FilterRTWStateStorageClass=Auto  ParallelPVariant=Passthrough  IdealPVariant=InternalParameters  IVariant=InternalParameters  DVariant=Disabled  IntegratorVariant=Continuous  SatVariant=Enabled  AWVariant=BackCalculation  PCopyVariant=Disabled  TRVariant=Disabled  FdbkBlocksVariant=Forward  IdealPFdbkVariant=Disabled  SatFdbkVariant=Disabled  DerivativeFilterVariant=Disabled  NVariant=Disabled  NCopyVariant=Disabled_SignalSpec  FilterICVariant=Disabled  IntegratorICVariant=InternalICs  ExternalResetVariant=Disabled  TRSumVariant=Passthrough  SumFdbkVariant=Disabled  SumVariant=Sum_PI  TsampFilterVariant=InternalTs  TsampNgainVariant=Passthrough  TsampIntegralVariant=Disabled_SignalSpec  ExternalSaturationOutDataTypeStr=Inherit: Same as second input  DerivativeSourceVariant=Disabled  PreIntVariant=InternalPreInt
  Sum : Sum  Inputs=|-+
  Transfer Fcn : TransferFcn  Denominator=[2 1]
  cmd : Outport
  wires:
  Transfer Fcn/1 -> Mux1/2, cmd/1
  T_set/1 -> Mux/1, Sum/1
  T_meas/1 -> Mux/2, Sum/2
  Sum/1 -> PID Controller/1
  PID Controller/1 -> Mux1/1, Transfer Fcn/1
  Mux/1 -> Control Signals/1
  Mux1/1 -> Control Signals/2

== system PEMFuelCellSystem_GasMixture_cEGR_RouteA_v2_v01/System_Control_Observability/Electrical Load/Inputs/Current Demand ==
  Current Demand : FromWorkspace  VariableName=[drive_cycle_time, drive_cycle_current]
  PS-Simulink Converter : nesl_utility/PS-Simulink Converter  PhysicalDomain=network_engine_domain  SubClassName=ps_output  LeftPortType=input  RightPortType=output  PseudoPeriodic=off  Frequencies=[]  VectorFormat=1-D array  Unit=V  AffineConversion=off
  Simulink-PS Converter : nesl_utility/Simulink-PS Converter  PhysicalDomain=network_engine_domain  SubClassName=ps_input  LeftPortType=input  RightPortType=output  PseudoPeriodic=off  Frequencies=[]  NoiseDistribution=none  NoiseParameters=[]  Unit=A  AffineConversion=off  FilteringAndDerivatives=provide  SimscapeFilterOrder=1  InputFilterTimeConstant=0.001  UdotUserProvided=0
  i : PMIOPort  Side=Left
  v : PMIOPort  Port=2  Side=Left
  tag scope: i_stack=global, v_stack=global
  wires:
  PS-Simulink Converter/1 -> [v_stack]
  Current Demand/1 -> [i_stack], Simulink-PS Converter/1  "routeA_current_profile_cmd_A"
  connections:
  Simulink-PS Converter/RConn1 -- i/RConn1
  PS-Simulink Converter/LConn1 -- v/RConn1

== system PEMFuelCellSystem_GasMixture_cEGR_RouteA_v2_v01/System_Control_Observability/Electrical Load/Inputs/Power Demand ==
  From Workspace : FromWorkspace  VariableName=[drive_cycle_time, drive_cycle_power]
  PS Divide : fl_lib/Physical Signals/Functions/PS Divide
  PS-Simulink Converter : nesl_utility/PS-Simulink Converter  PhysicalDomain=network_engine_domain  SubClassName=ps_output  LeftPortType=input  RightPortType=output  PseudoPeriodic=off  Frequencies=[]  VectorFormat=1-D array  Unit=V  AffineConversion=off
  PS-Simulink Converter1 : nesl_utility/PS-Simulink Converter  PhysicalDomain=network_engine_domain  SubClassName=ps_output  LeftPortType=input  RightPortType=output  PseudoPeriodic=off  Frequencies=[]  VectorFormat=1-D array  Unit=A  AffineConversion=off
  Power Current Limit : fl_lib/Physical Signals/Nonlinear Operators/PS Saturation  upper_limit=routeA_voltage_current_max_A A  lower_limit=routeA_voltage_current_min_A A  ZeroCross=true
  Power kW to W : Gain  Gain=1000
  Simulink-PS Converter : nesl_utility/Simulink-PS Converter  PhysicalDomain=network_engine_domain  SubClassName=ps_input  LeftPortType=input  RightPortType=output  PseudoPeriodic=off  Frequencies=[]  NoiseDistribution=none  NoiseParameters=[]  Unit=W  AffineConversion=off  FilteringAndDerivatives=provide  SimscapeFilterOrder=1  InputFilterTimeConstant=0.001  UdotUserProvided=0
  i : PMIOPort  Side=Left
  v : PMIOPort  Port=2  Side=Left
  tag scope: i_stack=global, v_stack=global
  wires:
  PS-Simulink Converter1/1 -> [i_stack]  "routeA_power_current_cmd_limited_A"
  PS-Simulink Converter/1 -> [v_stack]
  From Workspace/1 -> Power kW to W/1
  Power kW to W/1 -> Simulink-PS Converter/1
  connections:
  PS-Simulink Converter1/LConn1 -- Power Current Limit/RConn1 -- i/RConn1
  v/RConn1 -- PS-Simulink Converter/LConn1 -- PS Divide/LConn2
  PS Divide/LConn1 -- Simulink-PS Converter/RConn1
  PS Divide/RConn1 -- Power Current Limit/LConn1

== system PEMFuelCellSystem_GasMixture_cEGR_RouteA_v2_v01/System_Control_Observability/Electrical Load/Inputs/Voltage Demand ==
  Current Command : nesl_utility/Simulink-PS Converter  PhysicalDomain=network_engine_domain  SubClassName=ps_input  LeftPortType=input  RightPortType=output  PseudoPeriodic=off  Frequencies=[]  NoiseDistribution=none  NoiseParameters=[]  Unit=A  AffineConversion=off  FilteringAndDerivatives=provide  SimscapeFilterOrder=1  InputFilterTimeConstant=0.001  UdotUserProvided=0
  Current Command Dynamics : TransferFcn  Denominator=[0.1 1]
  Raw PI Diagnostic : slpidlib/PID Controller  Controller=PI  Form=Parallel  TimeDomain=Continuous-time  UseExternalTs=off  SampleTime=-1  IntegratorMethod=Forward Euler  FilterMethod=Forward Euler  ControllerParametersSource=internal  P=routeA_voltage_pi_Kp  I=routeA_voltage_pi_Ki  UseKiTs=off  D=0  UseExternalDerivativeSource=off  N=100  UseFilter=on  TunerSelectOption=Transfer Function Based (PID Tuner App)  InitialConditionSource=internal  InitialConditionForIntegrator=0  InitialConditionForFilter=0  DifferentiatorICPrevScaledInput=0  ExternalReset=none  TrackingMode=off  Kt=1  LimitOutput=off  SatLimitsSource=internal  UpperSaturationLimit=inf  LowerSaturationLimit=-inf  LinearizeAsGain=on  AntiWindupMode=none  Kb=1  LimitIntegrator=off  UpperIntegratorSaturationLimit=inf  LowerIntegratorSaturationLimit=-inf  POutMin=[]  POutMax=[]  IOutMin=[]  IOutMax=[]  DOutMin=[]  DOutMax=[]  NOutMin=[]  NOutMax=[]  SumOutMin=[]  SumOutMax=[]  SaturationOutMin=[]  SaturationOutMax=[]  PParamMin=[]  PParamMax=[]  IParamMin=[]  IParamMax=[]  DParamMin=[]  DParamMax=[]  NParamMin=[]  NParamMax=[]  KbParamMin=[]  KbParamMax=[]  KtParamMin=[]  KtParamMax=[]  KbOutMin=[]  KbOutMax=[]  KtOutMin=[]  KtOutMax=[]  IntegratorOutMin=[]  IntegratorOutMax=[]  FilterOutMin=[]  FilterOutMax=[]  SumI1OutMin=[]  SumI1OutMax=[]  SumI2OutMin=[]  SumI2OutMax=[]  SumI3OutMin=[]  SumI3OutMax=[]  SumI4OutMin=[]  SumI4OutMax=[]  SumDOutMin=[]  SumDOutMax=[]  DifferentiatorOutMin=[]  DifferentiatorOutMax=[]  FilterDiffOutCoefMin=[]  FilterDiffOutCoefMax=[]  ReciprocalOutMin=[]  ReciprocalOutMax=[]  SumDenOutMin=[]  SumDenOutMax=[]  SumNumOutMin=[]  SumNumOutMax=[]  DivideOutMin=[]  DivideOutMax=[]  UdiffTsProdOutMin=[]  UdiffTsProdOutMax=[]  NTsProdOutMin=[]  NTsProdOutMax=[]  UintegralTsProdOutMin=[]  UintegralTsProdOutMax=[]  UngainTsProdOutMin=[]  UngainTsProdOutMax=[]  ClampingZeroOutDataTypeStr=Inherit: Inherit via back propagation  ClampingZeroOutMin=[]  ClampingZeroOutMax=[]  FilterDenConstantOutDataTypeStr=Inherit: Inherit via back propagation  FilterDenConstantOutMin=[]  FilterDenConstantOutMax=[]  PCopyOutDataTypeStr=Inherit: Inherit via back propagation  PCopyOutMin=[]  PCopyOutMax=[]  NCopyOutDataTypeStr=Inherit: Inherit via back propagation  NCopyOutMin=[]  NCopyOutMax=[]  IntegratorContinuousStateAttributes=''  IntegratorStateMustResolveToSignalObject=off  IntegratorRTWStateStorageClass=Auto  FilterContinuousStateAttributes=''  FilterStateMustResolveToSignalObject=off  FilterRTWStateStorageClass=Auto  ParallelPVariant=InternalParameters  IdealPVariant=Disabled  IVariant=InternalParameters  DVariant=Disabled  IntegratorVariant=Continuous  SatVariant=Disabled  AWVariant=Passthrough  PCopyVariant=Disabled  TRVariant=Disabled  FdbkBlocksVariant=Forward  IdealPFdbkVariant=Disabled  SatFdbkVariant=Disabled  DerivativeFilterVariant=Disabled  NVariant=Disabled  NCopyVariant=Disabled_SignalSpec  FilterICVariant=Disabled  IntegratorICVariant=InternalICs  ExternalResetVariant=Disabled  TRSumVariant=Passthrough  SumFdbkVariant=Disabled  SumVariant=Sum_PI  TsampFilterVariant=InternalTs  TsampNgainVariant=Passthrough  TsampIntegralVariant=Disabled_SignalSpec  ExternalSaturationOutDataTypeStr=Inherit: Same as second input  DerivativeSourceVariant=Disabled  PreIntVariant=InternalPreInt
  Saturation Status : RelationalOperator  Operator=~=
  Saturation Status Terminator : Terminator
  Voltage Error : Sum  Inputs=+-
  Voltage Measurement : nesl_utility/PS-Simulink Converter  PhysicalDomain=network_engine_domain  SubClassName=ps_output  LeftPortType=input  RightPortType=output  PseudoPeriodic=off  Frequencies=[]  VectorFormat=inherit  Unit=V  AffineConversion=off
  Voltage PI : slpidlib/PID Controller  Controller=PI  Form=Parallel  TimeDomain=Continuous-time  UseExternalTs=off  SampleTime=-1  IntegratorMethod=Forward Euler  FilterMethod=Forward Euler  ControllerParametersSource=internal  P=routeA_voltage_pi_Kp  I=routeA_voltage_pi_Ki  UseKiTs=off  D=0  UseExternalDerivativeSource=off  N=100  UseFilter=on  TunerSelectOption=Transfer Function Based (PID Tuner App)  InitialConditionSource=internal  InitialConditionForIntegrator=0  InitialConditionForFilter=0  DifferentiatorICPrevScaledInput=0  ExternalReset=none  TrackingMode=off  Kt=1  LimitOutput=on  SatLimitsSource=internal  UpperSaturationLimit=routeA_voltage_current_max_A  LowerSaturationLimit=routeA_voltage_current_min_A  LinearizeAsGain=on  AntiWindupMode=clamping  Kb=1  LimitIntegrator=off  UpperIntegratorSaturationLimit=inf  LowerIntegratorSaturationLimit=-inf  POutMin=[]  POutMax=[]  IOutMin=[]  IOutMax=[]  DOutMin=[]  DOutMax=[]  NOutMin=[]  NOutMax=[]  SumOutMin=[]  SumOutMax=[]  SaturationOutMin=[]  SaturationOutMax=[]  PParamMin=[]  PParamMax=[]  IParamMin=[]  IParamMax=[]  DParamMin=[]  DParamMax=[]  NParamMin=[]  NParamMax=[]  KbParamMin=[]  KbParamMax=[]  KtParamMin=[]  KtParamMax=[]  KbOutMin=[]  KbOutMax=[]  KtOutMin=[]  KtOutMax=[]  IntegratorOutMin=[]  IntegratorOutMax=[]  FilterOutMin=[]  FilterOutMax=[]  SumI1OutMin=[]  SumI1OutMax=[]  SumI2OutMin=[]  SumI2OutMax=[]  SumI3OutMin=[]  SumI3OutMax=[]  SumI4OutMin=[]  SumI4OutMax=[]  SumDOutMin=[]  SumDOutMax=[]  DifferentiatorOutMin=[]  DifferentiatorOutMax=[]  FilterDiffOutCoefMin=[]  FilterDiffOutCoefMax=[]  ReciprocalOutMin=[]  ReciprocalOutMax=[]  SumDenOutMin=[]  SumDenOutMax=[]  SumNumOutMin=[]  SumNumOutMax=[]  DivideOutMin=[]  DivideOutMax=[]  UdiffTsProdOutMin=[]  UdiffTsProdOutMax=[]  NTsProdOutMin=[]  NTsProdOutMax=[]  UintegralTsProdOutMin=[]  UintegralTsProdOutMax=[]  UngainTsProdOutMin=[]  UngainTsProdOutMax=[]  ClampingZeroOutDataTypeStr=Inherit: Inherit via back propagation  ClampingZeroOutMin=[]  ClampingZeroOutMax=[]  FilterDenConstantOutDataTypeStr=Inherit: Inherit via back propagation  FilterDenConstantOutMin=[]  FilterDenConstantOutMax=[]  PCopyOutDataTypeStr=Inherit: Inherit via back propagation  PCopyOutMin=[]  PCopyOutMax=[]  NCopyOutDataTypeStr=Inherit: Inherit via back propagation  NCopyOutMin=[]  NCopyOutMax=[]  IntegratorContinuousStateAttributes=''  IntegratorStateMustResolveToSignalObject=off  IntegratorRTWStateStorageClass=Auto  FilterContinuousStateAttributes=''  FilterStateMustResolveToSignalObject=off  FilterRTWStateStorageClass=Auto  ParallelPVariant=InternalParameters  IdealPVariant=Disabled  IVariant=InternalParameters  DVariant=Disabled  IntegratorVariant=Continuous  SatVariant=Enabled  AWVariant=ContClampingParallel  PCopyVariant=Disabled  TRVariant=Disabled  FdbkBlocksVariant=Forward  IdealPFdbkVariant=Disabled  SatFdbkVariant=Disabled  DerivativeFilterVariant=Disabled  NVariant=Disabled  NCopyVariant=Disabled_SignalSpec  FilterICVariant=Disabled  IntegratorICVariant=InternalICs  ExternalResetVariant=Disabled  TRSumVariant=Passthrough  SumFdbkVariant=Disabled  SumVariant=Sum_PI  TsampFilterVariant=InternalTs  TsampNgainVariant=Passthrough  TsampIntegralVariant=Disabled_SignalSpec  ExternalSaturationOutDataTypeStr=Inherit: Same as second input  DerivativeSourceVariant=Disabled  PreIntVariant=InternalPreInt
  Voltage Reference : FromWorkspace  VariableName=[drive_cycle_time, drive_cycle_voltage]
  i : PMIOPort  Side=Left
  v : PMIOPort  Port=2  Side=Left
  tag scope: i_stack=global, v_stack=global
  wires:
  Current Command Dynamics/1 -> [i_stack], Current Command/1  "routeA_voltage_current_cmd_A"
  Voltage PI/1 -> Current Command Dynamics/1, Saturation Status/2  "routeA_voltage_current_cmd_limited_A"
  Voltage Error/1 -> Raw PI Diagnostic/1, Voltage PI/1  "routeA_voltage_control_error_V"
  Voltage Reference/1 -> Voltage Error/2  "routeA_voltage_ref_V"
  Voltage Measurement/1 -> Voltage Error/1, [v_stack]
  Raw PI Diagnostic/1 -> Saturation Status/1  "routeA_voltage_current_cmd_raw_A"
  Saturation Status/1 -> Saturation Status Terminator/1  "routeA_voltage_current_saturated"
  connections:
  v/RConn1 -- Voltage Measurement/LConn1
  Current Command/RConn1 -- i/RConn1

== matlab function PEMFuelCellSystem_GasMixture_cEGR_RouteA_v2_v01/Cathode_Exhaust_Backpressure_Water/SeparatorOrCondensation ==
  data: p_MPa input; m_water_sep output; T_degC input; y_i input; egr_mdot input; exhaust_mdot input
function m_water_sep = SeparatorOrCondensation(p_MPa,T_degC,y_i,egr_mdot,exhaust_mdot)
%#codegen
% L2 saturation-excess estimator. Source: l2_saturation_excess_estimator.
p = max(double(p_MPa), 1e-6);
T = double(T_degC);
if T > 200
    Tc = T - 273.15;
else
    Tc = T;
end
Tc = min(max(Tc, -40), 120);
if numel(y_i) >= 4
    yH2O = max(double(y_i(4)), 0);
else
    yH2O = 0;
end
pSat_kPa = 0.61121 * exp((18.678 - Tc/234.5) * (Tc/(257.14 + Tc)));
pSat_MPa = max(pSat_kPa * 1e-3, 1e-9);
ySat = min(max(pSat_MPa / p, 0), 1);
excess = max(yH2O - ySat, 0);
mdotTotal = max(double(egr_mdot), 0) + max(double(exhaust_mdot), 0);
m_water_sep = mdotTotal * excess;
end
